simulink model "direct_form_I"  (R2015a)
settings: Solver=ode45  StartTime=0.0  StopTime=10.0  RelTol=1e-3
undefined symbols (not defined in the file): sml_a1, sml_a2, sml_b0, sml_b1, sml_b2, sml_initial_states, sml_input_const, sml_prec_frac, sml_prec_int
libraries: simulink x1
settings Model: PauseTimes=4  SnapshotBufferSize=4  SnapshotInterval=4  Creator=Lennon  LastModifiedBy=lennon
settings DebuggingCC: ParameterOverflowMsg=none  ParameterPrecisionLossMsg=none  ParameterTunabilityLossMsg=none

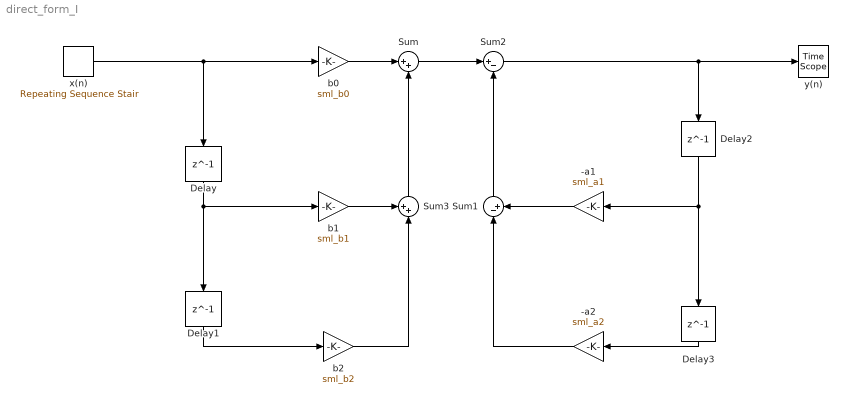
== system direct_form_I ==
  -a1 : Gain  Gain=sml_a1  ParamDataTypeStr=fixdt(1,sml_prec_int+sml_prec_frac,sml_prec_frac)  OutDataTypeStr=fixdt(1,sml_prec_int+sml_prec_frac,sml_prec_frac)  RndMeth=Round
  -a2 : Gain  Gain=sml_a2  ParamDataTypeStr=fixdt(1,sml_prec_int+sml_prec_frac,sml_prec_frac)  OutMin=0  OutDataTypeStr=fixdt(1,sml_prec_int+sml_prec_frac,sml_prec_frac)  RndMeth=Round
  Delay : Delay  DelayLength=1  InitialCondition=sml_input_const  InputProcessing=Inherited  SampleTime=1
  Delay1 : Delay  DelayLength=1  InitialCondition=sml_input_const  SampleTime=1
  Delay2 : Delay  DelayLength=1  InitialCondition=norm(sml_initial_states)  SampleTime=1
  Delay3 : Delay  DelayLength=1  InitialCondition=norm(sml_initial_states)  SampleTime=1
  Sum : Sum  Inputs=|++  AccumDataTypeStr=fixdt(1,sml_prec_int+sml_prec_frac,sml_prec_frac)  OutDataTypeStr=fixdt(1,sml_prec_int+sml_prec_frac,sml_prec_frac)  RndMeth=Round
  Sum1 : Sum  Inputs=|-+  AccumDataTypeStr=fixdt(1,sml_prec_int+sml_prec_frac,sml_prec_frac)  OutDataTypeStr=fixdt(1,sml_prec_int+sml_prec_frac,sml_prec_frac)  RndMeth=Round
  Sum2 : Sum  Inputs=|+-  AccumDataTypeStr=fixdt(1,sml_prec_int+sml_prec_frac,sml_prec_frac)  OutDataTypeStr=fixdt(1,sml_prec_int+sml_prec_frac,sml_prec_frac)  RndMeth=Round
  Sum3 : Sum  Inputs=++|  AccumDataTypeStr=fixdt(1,sml_prec_int+sml_prec_frac,sml_prec_frac)  OutDataTypeStr=fixdt(1,sml_prec_int+sml_prec_frac,sml_prec_frac)  RndMeth=Round
  b0 : Gain  Gain=sml_b0  ParamDataTypeStr=fixdt(1,sml_prec_int+sml_prec_frac,sml_prec_frac)  OutDataTypeStr=fixdt(1,sml_prec_int+sml_prec_frac,sml_prec_frac)  RndMeth=Round
  b1 : Gain  Gain=sml_b1  ParamDataTypeStr=fixdt(1,sml_prec_int+sml_prec_frac,sml_prec_frac)  OutDataTypeStr=fixdt(1,sml_prec_int+sml_prec_frac,sml_prec_frac)  RndMeth=Round
  b2 : Gain  Gain=sml_b2  ParamDataTypeStr=fixdt(1,sml_prec_int+sml_prec_frac,sml_prec_frac)  OutDataTypeStr=fixdt(1,sml_prec_int+sml_prec_frac,sml_prec_frac)  RndMeth=Round
  x(n) : simulink/Sources/Repeating Sequence Stair  OutValues=[sml_input_const sml_input_const sml_input_const sml_input_const sml_input_const sml_input_const sml_input_const sml_input_const sml_input_const sml_input_const]  tsamp=1  OutMin=[]  OutMax=[]  OutDataTypeStr=fixdt(1,sml_prec_int+sml_prec_frac,sml_prec_frac)  OutputDataTypeScalingMode=Specify via dialog  OutDataType=fixdt(1,sml_prec_int+sml_prec_frac,sml_prec_frac)  ConRadixGroup=Best Precision: Vector-wise  OutScaling=[]
  y(n) : TimeScope
  wires:
  Delay/1 -> Delay1/1, b1/1
  b0/1 -> Sum/1
  Sum/1 -> Sum2/1
  Sum2/1 -> Delay2/1, y(n)/1
  x(n)/1 -> Delay/1, b0/1
  Delay1/1 -> b2/1
  Delay3/1 -> -a2/1
  Delay2/1 -> -a1/1, Delay3/1
  b1/1 -> Sum3/1
  Sum3/1 -> Sum/2
  b2/1 -> Sum3/2
  -a2/1 -> Sum1/1
  -a1/1 -> Sum1/2
  Sum1/1 -> Sum2/2
